simulink model "ball_table"  (R2015a)
settings: Solver=ode45  StartTime=0.0  StopTime=50  RelTol=1e-3
InitFcn:
  | B=0.1
  | M=0.5
  | g=10
settings Model: Creator=PC  LastModifiedBy=PC

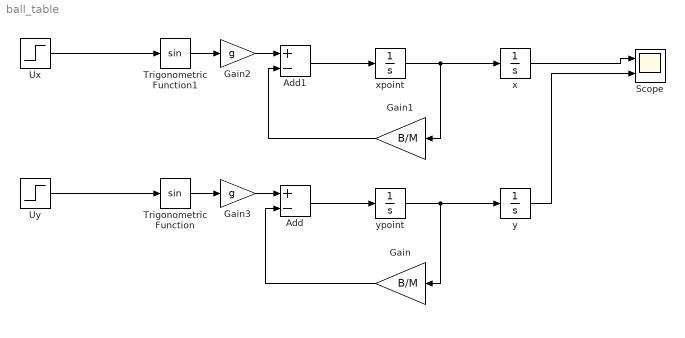
== system ball_table ==
  Add : Sum  Inputs=+-
  Add1 : Sum  Inputs=+-
  Gain : Gain  Gain=B/M
  Gain1 : Gain  Gain=B/M
  Gain2 : Gain  Gain=g
  Gain3 : Gain  Gain=g
  Scope : Scope  NumInputPorts=2
      settings: YMin=-5~-5  YMax=5~5
  Trigonometric Function : Trigonometry
  Trigonometric Function1 : Trigonometry
  Ux : Step  After=0  SampleTime=0
  Uy : Step  After=0  SampleTime=0
  x : Integrator
  xpoint : Integrator
  y : Integrator
  ypoint : Integrator
  wires:
  Gain2/1 -> Add1/1
  Trigonometric Function1/1 -> Gain2/1
  Gain3/1 -> Add/1
  Trigonometric Function/1 -> Gain3/1
  Gain/1 -> Add/2
  Gain1/1 -> Add1/2
  Add1/1 -> xpoint/1
  xpoint/1 -> x/1, Gain1/1
  Add/1 -> ypoint/1
  ypoint/1 -> y/1, Gain/1
  x/1 -> Scope/1
  y/1 -> Scope/2
  Ux/1 -> Trigonometric Function1/1
  Uy/1 -> Trigonometric Function/1
